simulink model "Seri_HEV_Model"  (R2025b)
(part 3 of 4)

  Ön Tekerlek : sdl_lib/Tires & Vehicles/Tire (Magic Formula)  parameterization=sdl.enum.magic_tire_model.peak  F_z1=3000 N  F_x1=3500 N  kappa1=10  B_m=10  C_m=1.9  D_m=1  E_m=0.97  fz0=4000 N  p_Cx=1.685  p_Dx=[1.21, -.037]  p_Ex=[.344, .095, -.02, 0]  p_Kx=[21.51, -.163, .245]  p_Hx=[-.002, .002]  p_Vx=[0, 0]  rolling_radius_model=sdl.enum.RollingRadiusParameterization.Constant  r_e=Wheel_Radius m  r_0=0.3 m  breff=8.39  dreff=0.26  freff=0.074  q_re0=0.99  q_v1=0.008  longvl=17 m/s  cz=5e5 N/m  model_resistance=false  resistance_model=sdl.enum.rollingResistanceParameterization.constant  coeff=0.015  p_tire=250e3 Pa  alpha=-0.003  beta=0.97  coeff_a=84e-4  coeff_b=6.2e-4 s/m  coeff_c=1.6e-4 s^2/m^2  p_tire0=240e3 Pa  fz0_resistance=4000 N  vH0=16 m/s  q_Sy=[.0082, 0, .0014, .001, 0, 0, 1.08, -.5]  v_thr=0.001 m/s  enable_scaling_coefficients=false  lfzO=1  lcx=1  lmux=1  lex=1  lkx=1  lhx=1  lvx=1  lmy=1  model_compliance=sdl.enum.compliance.off  stiffness=1e6 N/m  damping=1000 N*s/m  model_inertia=sdl.enum.model_inertia.off  inertia=1 kg*m^2  initial_velocity=0 rad/s  vxlow=1 m/s  v_tr_thr=0.1 m/s  kpumin=-1.5  kpumax=1.5
  Hiz : Outport
  BattSoc : Outport  Port=2
  CO2 Emisyonu : Outport  Port=3
  Yakit Tuketimi : Outport  Port=4
  wires:
  Datasheet Battery/1 -> Bus Selector/1
  Longitudinal Driver/3 -> Kontrolcü/1(Decel)
  Mapped SI Engine/1 -> Bus Selector1/1
  Drive Cycle Source/1 -> Longitudinal Driver/1
  Integrator3/1 -> BattSoc/1
  Longitudinal Driver/1 -> Terminator2/1
  Mapped Motor/1 -> Terminator/1
  Longitudinal Driver/2 -> Kontrolcü/2(Accel)
  Gain1/1 -> Hiz/1  "Hiz"
  Bus Selector/1 -> Integrator3/1, Kontrolcü/3(SOC)  "<BattSoc>"
  Constant1/1 -> Datasheet Battery/2
  Grade/1 -> Longitudinal Driver/3
  Constant/1 -> Generatör/2, Mapped SI Engine/2  "Benzinli_Motor_Devri"
  Generatör/3 -> Terminator1/1
  Generatör/2 -> Add/2  "Jenerator_Akimi"
  Mapped Motor/2 -> Add/1  "Ana_Motor_Akimi"
  Add/1 -> Unit Delay3/1
  Unit Delay3/1 -> Datasheet Battery/1
  Datasheet Battery/2 -> Mapped Motor/1, Generatör/1  "Batarya_Durumu"
  Kontrolcü/2(Trq_ICE) -> Mapped SI Engine/1
  PS-Simulink Converter/1 -> Integrator/1, Longitudinal Driver/2, Unit Delay4/1
  Unit Delay4/1 -> Gain/1, Gain1/1, Kontrolcü/4(V)
  Integrator/1 -> Gain2/1
  Integrator1/1 -> Gain3/1
  Bus Selector1/1 -> Integrator1/1  "<FuelMassFlw>"
  Gain2/1 -> Divide1/2, Divide/2  "Hiz"
  Integrator2/1 -> Gain4/1
  Bus Selector1/2 -> Integrator2/1  "<EoCO2>"
  Divide1/1 -> CO2 Emisyonu/1  "CO2 Emisyonu"
  Divide/1 -> Yakit Tuketimi/1  "Yakit Tuketimi"
  Mapped SI Engine/2 -> Gain5/1
  Gain5/1 -> Generatör/3  "Hiz"
  Kontrolcü/1(Trq_EM) -> Mapped Motor/3, Simulink-PS Converter/1
  Mapped Motor/3 -> Terminator3/1
  Gain/1 -> Mapped Motor/2
  Gain3/1 -> Divide/1  "fuel"
  Gain4/1 -> Divide1/1  "eoCo2"
  connections:
  PS Terminator/LConn1 -- Ön Tekerlek/RConn1
  PS Constant/RConn1 -- Vehicle Body/LConn3
  Vehicle Body/LConn1 -- Arka Tekerlek/RConn2 -- Solver Configuration/RConn1 -- Ön Tekerlek/RConn2
  Simple Gear/RConn1 -- Arka Tekerlek/LConn2 -- Ön Tekerlek/LConn2
  PS Terminator1/LConn1 -- Arka Tekerlek/RConn1
  Vehicle Body/RConn1 -- Arka Tekerlek/LConn1
  PS Constant1/RConn1 -- Vehicle Body/RConn3
  Ön Tekerlek/LConn1 -- Vehicle Body/RConn2
  Mechanical Rotational Reference/LConn1 -- Ideal Torque Source/RConn2
  Ideal Torque Source/LConn1 -- Simple Gear/LConn1
  Simulink-PS Converter/RConn1 -- Ideal Torque Source/RConn1
  Vehicle Body/LConn2 -- PS-Simulink Converter/LConn1
